simulink model "CE1"  (R2023b)
settings: Solver=VariableStepAuto  StartTime=0.0  StopTime=499.75  RelTol=1e-3
values from neighbouring files (symbols this model uses):
  Ts = 0.25    [CE1_1.m]    (also in CE1_3.m; CE1_4.m; CE1_5.m; CE1_6.m)
settings Model: Creator=jules  LastModifiedBy=maxim

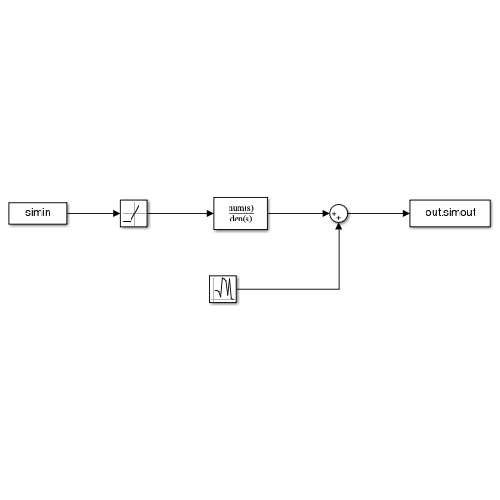
[thumbnail: Simulink's stored preview of the top-level diagram]
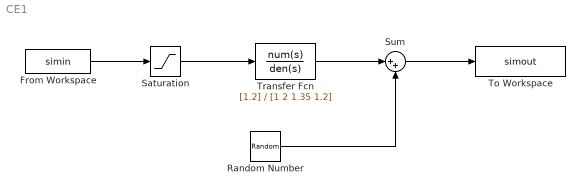
== system CE1 ==
  From Workspace : FromWorkspace  VariableName=simin  SampleTime=Ts
  Random Number : RandomNumber  Variance=0.01  SampleTime=Ts
  Saturation : Saturate  UpperLimit=0.7  LowerLimit=-0.7
  Sum : Sum  Inputs=|++
  To Workspace : ToWorkspace  VariableName=simout  SaveFormat=Timeseries  SampleTime=Ts
  Transfer Fcn : TransferFcn  Numerator=[1.2]  Denominator=[1 2 1.35 1.2]
  wires:
  Saturation/1 -> Transfer Fcn/1
  From Workspace/1 -> Saturation/1
  Sum/1 -> To Workspace/1
  Transfer Fcn/1 -> Sum/1
  Random Number/1 -> Sum/2
